simulink model "model2_unstable__lqr_controller_observer"  (R2022b)
settings: Solver=VariableStepAuto  StartTime=0.0  StopTime=10  RelTol=1e-3
InitFcn:
  | model2_init_params_unstable__lqr_controller
values from neighbouring files (symbols this model uses):
  A = [ ... (first row only)    [model1_init_params_stable.m]    (also in model1_init_params_unstable.m; model2_init_params_stable.m; model2_init_params_unstable.m; model2_init_params_unstable__lqr_controller.m)
  A_ccf = [ ... (first row only)    [model2_init_params_stable.m]    (also in model2_init_params_unstable.m; model2_init_params_unstable__lqr_controller.m)
  A_obs = A-L*C    [model1_init_params_stable.m]    (also in model1_init_params_unstable.m; model2_init_params_unstable__lqr_controller.m = A_ccf-L*C_ccf)
  B = [ ... (first row only)    [model1_init_params_stable.m]    (also in model1_init_params_unstable.m; model2_init_params_stable.m; model2_init_params_unstable.m; model2_init_params_unstable__lqr_controller.m)
  B_obs = [B L]    [model1_init_params_stable.m]    (also in model1_init_params_unstable.m; model2_init_params_unstable__lqr_controller.m = [B_ccf L])
  C = [(V^2*h-a*c*g)*sin(lambda)/(b*h^2)*k1 a*V*sin(lambda)/(b*h)*k1]    [model1_init_params_stable.m]    (also in model1_init_params_unstable.m; model2_init_params_stable.m = [1 0 0 0]; model2_init_params_unstable.m = [1 0 0 0]; model2_init_params_unstable__lqr_controller.m = [1 0 0 0])
  C_ccf = [tf_num(5)  tf_num(4)   tf_num(3)   tf_num(2)]    [model2_init_params_stable.m]    (also in model2_init_params_unstable.m; model2_init_params_unstable__lqr_controller.m)
  C_obs = eye(length(A_obs))    [model1_init_params_stable.m]    (also in model1_init_params_unstable.m; model2_init_params_unstable__lqr_controller.m)
  D = 0    [model1_init_params_stable.m]    (also in model1_init_params_unstable.m; model2_init_params_stable.m; model2_init_params_unstable.m; model2_init_params_unstable__lqr_controller.m)
  D_obs = zeros(size(B_obs))    [model1_init_params_stable.m]    (also in model1_init_params_unstable.m; model2_init_params_unstable__lqr_controller.m)
  K = place(A,B,new_poles)    [model1_init_params_unstable.m]    (also in model2_init_params_unstable.m = place(A_ccf,B_ccf,new_poles))
settings Model: Creator=neotod  LastModifiedBy=neotod

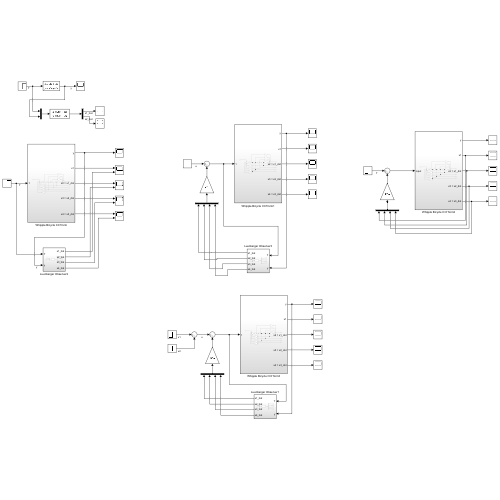
[thumbnail: Simulink's stored preview of the top-level diagram]
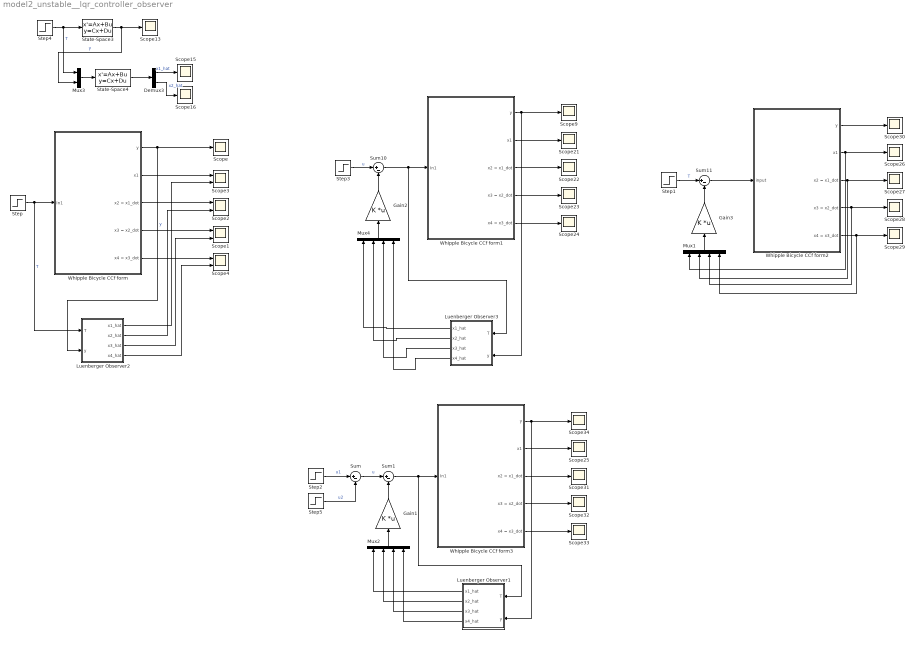
== system model2_unstable__lqr_controller_observer ==
  Demux3 : Demux  Outputs=2
  Gain1 : Gain  Gain=K  Multiplication=Matrix(K*u)
  Gain2 : Gain  Gain=K  Multiplication=Matrix(K*u)
  Gain3 : Gain  Gain=K  Multiplication=Matrix(K*u)
  Luenberger Observer1 : Subsystem
  Luenberger Observer2 : Subsystem
  Luenberger Observer3 : Subsystem
  Mux1 : Mux
  Mux2 : Mux
  Mux3 : Mux  Inputs=2
  Mux4 : Mux
  Scope{,9,13,15..16,21..34} (19 alike) : Scope
  Scope{1..4} (4 alike) : Scope  NumInputPorts=2
  State-Space3 : StateSpace  A=A  B=B  C=C  D=D  InitialCondition=0
  State-Space4 : StateSpace  A=A_obs  B=B_obs  C=C_obs  D=D_obs  InitialCondition=0
  Step : Step  After=0.6  SampleTime=0
  Step1 : Step  After=0.6  SampleTime=0
  Step2 : Step  Time=0.25  SampleTime=0
  Step3 : Step  After=0.6  SampleTime=0
  Step4 : Step  SampleTime=0
  Step5 : Step  Time=0.5  SampleTime=0
  Sum{,1,10..11} (4 alike) : Sum  Inputs=|+-
  Whipple Bicycle CCf form : Subsystem
  Whipple Bicycle CCf form1 : Subsystem
  Whipple Bicycle CCf form2 : Subsystem
  Whipple Bicycle CCf form3 : Subsystem
  wires:
  Step4/1 -> Mux3/1, State-Space3/1  "T"
  State-Space3/1 -> Mux3/2, Scope13/1  "y"
  State-Space4/1 -> Demux3/1
  Mux3/1 -> State-Space4/1
  Demux3/1 -> Scope15/1  "x1_hat"
  Demux3/2 -> Scope16/1  "x2_hat"
  Whipple Bicycle CCf form/2(x1) -> Scope3/1
  Whipple Bicycle CCf form/5(x4 = x3_dot) -> Scope4/1
  Whipple Bicycle CCf form/4(x3 = x2_dot) -> Scope1/1
  Whipple Bicycle CCf form/3(x2 = x1_dot) -> Scope2/1
  Step/1 -> Luenberger Observer2/1(T), Whipple Bicycle CCf form/1(In1)  "T"
  Whipple Bicycle CCf form/1(y) -> Luenberger Observer2/2(y), Scope/1  "y"
  Whipple Bicycle CCf form1/5(x4 = x3_dot) -> Scope24/1
  Luenberger Observer3/2(x2_hat) -> Mux4/2
  Whipple Bicycle CCf form1/4(x3 = x2_dot) -> Scope23/1
  Luenberger Observer3/3(x3_hat) -> Mux4/3
  Whipple Bicycle CCf form1/2(x1) -> Scope21/1
  Whipple Bicycle CCf form1/3(x2 = x1_dot) -> Scope22/1
  Luenberger Observer3/1(x1_hat) -> Mux4/1
  Luenberger Observer3/4(x4_hat) -> Mux4/4
  Whipple Bicycle CCf form1/1(y) -> Luenberger Observer3/2(y), Scope9/1
  Step3/1 -> Sum10/1  "u"
  Sum10/1 -> Luenberger Observer3/1(T), Whipple Bicycle CCf form1/1(In1)
  Mux4/1 -> Gain2/1
  Gain2/1 -> Sum10/2
  Sum11/1 -> Whipple Bicycle CCf form2/1(input)
  Step1/1 -> Sum11/1  "T"
  Whipple Bicycle CCf form2/2(x1) -> Mux1/1, Scope26/1
  Whipple Bicycle CCf form2/3(x2 = x1_dot) -> Mux1/2, Scope27/1
  Whipple Bicycle CCf form2/5(x4 = x3_dot) -> Mux1/4, Scope29/1
  Mux1/1 -> Gain3/1
  Gain3/1 -> Sum11/2
  Whipple Bicycle CCf form2/4(x3 = x2_dot) -> Mux1/3, Scope28/1
  Whipple Bicycle CCf form2/1(y) -> Scope30/1
  Sum1/1 -> Luenberger Observer1/1(T), Whipple Bicycle CCf form3/1(In1)
  Gain1/1 -> Sum1/2
  Whipple Bicycle CCf form3/4(x3 = x2_dot) -> Scope32/1
  Whipple Bicycle CCf form3/3(x2 = x1_dot) -> Scope31/1
  Whipple Bicycle CCf form3/1(y) -> Luenberger Observer1/2(y), Scope34/1
  Mux2/1 -> Gain1/1
  Luenberger Observer1/4(x4_hat) -> Mux2/4
  Luenberger Observer1/1(x1_hat) -> Mux2/1
  Whipple Bicycle CCf form3/5(x4 = x3_dot) -> Scope33/1
  Luenberger Observer1/2(x2_hat) -> Mux2/2
  Luenberger Observer1/3(x3_hat) -> Mux2/3
  Whipple Bicycle CCf form3/2(x1) -> Scope25/1
  Sum/1 -> Sum1/1  "u"
  Step2/1 -> Sum/1  "u1"
  Step5/1 -> Sum/2  "u2"
  Luenberger Observer2/1(x1_hat) -> Scope3/2
  Luenberger Observer2/2(x2_hat) -> Scope2/2
  Luenberger Observer2/3(x3_hat) -> Scope1/2
  Luenberger Observer2/4(x4_hat) -> Scope4/2

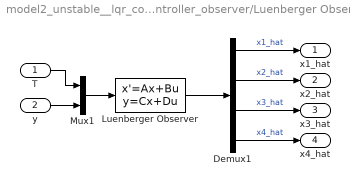
== system model2_unstable__lqr_controller_observer/Luenberger Observer1 ==
  T : Inport
  y : Inport  Port=2
  Demux1 : Demux
  Luenberger Observer : StateSpace  A=A_obs  B=B_obs  C=C_obs  D=D_obs  InitialCondition=0
  Mux1 : Mux  Inputs=2
  x1_hat : Outport
  x2_hat : Outport  Port=2
  x3_hat : Outport  Port=3
  x4_hat : Outport  Port=4
  wires:
  Demux1/2 -> x2_hat/1  "x2_hat"
  Mux1/1 -> Luenberger Observer/1
  Luenberger Observer/1 -> Demux1/1
  Demux1/1 -> x1_hat/1  "x1_hat"
  Demux1/3 -> x3_hat/1  "x3_hat"
  Demux1/4 -> x4_hat/1  "x4_hat"
  y/1 -> Mux1/2
  T/1 -> Mux1/1

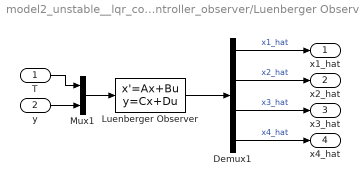
== system model2_unstable__lqr_controller_observer/Luenberger Observer2 ==
  T : Inport
  y : Inport  Port=2
  Demux1 : Demux
  Luenberger Observer : StateSpace  A=A_obs  B=B_obs  C=C_obs  D=D_obs  InitialCondition=0
  Mux1 : Mux  Inputs=2
  x1_hat : Outport
  x2_hat : Outport  Port=2
  x3_hat : Outport  Port=3
  x4_hat : Outport  Port=4
  wires:
  Demux1/2 -> x2_hat/1  "x2_hat"
  Mux1/1 -> Luenberger Observer/1
  Luenberger Observer/1 -> Demux1/1
  Demux1/1 -> x1_hat/1  "x1_hat"
  Demux1/3 -> x3_hat/1  "x3_hat"
  Demux1/4 -> x4_hat/1  "x4_hat"
  T/1 -> Mux1/1
  y/1 -> Mux1/2

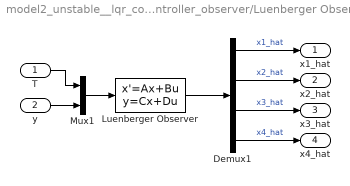
== system model2_unstable__lqr_controller_observer/Luenberger Observer3 ==
  T : Inport
  y : Inport  Port=2
  Demux1 : Demux
  Luenberger Observer : StateSpace  A=A_obs  B=B_obs  C=C_obs  D=D_obs  InitialCondition=0
  Mux1 : Mux  Inputs=2
  x1_hat : Outport
  x2_hat : Outport  Port=2
  x3_hat : Outport  Port=3
  x4_hat : Outport  Port=4
  wires:
  Demux1/2 -> x2_hat/1  "x2_hat"
  Mux1/1 -> Luenberger Observer/1
  Luenberger Observer/1 -> Demux1/1
  Demux1/1 -> x1_hat/1  "x1_hat"
  Demux1/3 -> x3_hat/1  "x3_hat"
  Demux1/4 -> x4_hat/1  "x4_hat"
  y/1 -> Mux1/2
  T/1 -> Mux1/1

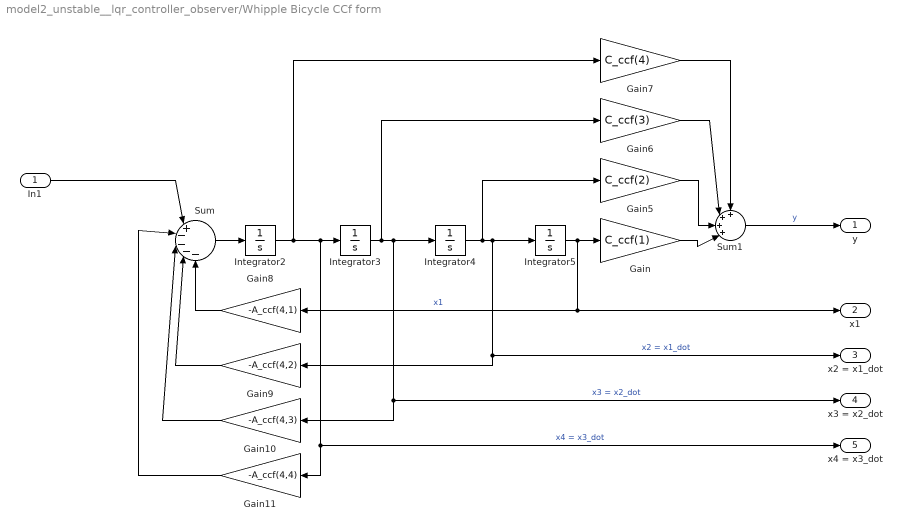
== system model2_unstable__lqr_controller_observer/Whipple Bicycle CCf form ==
  In1 : Inport
  Gain : Gain  Gain=C_ccf(1)
  Gain10 : Gain  Gain=-A_ccf(4,3)
  Gain11 : Gain  Gain=-A_ccf(4,4)
  Gain5 : Gain  Gain=C_ccf(2)
  Gain6 : Gain  Gain=C_ccf(3)
  Gain7 : Gain  Gain=C_ccf(4)
  Gain8 : Gain  Gain=-A_ccf(4,1)
  Gain9 : Gain  Gain=-A_ccf(4,2)
  Integrator{2..5} (4 alike) : Integrator
  Sum : Sum  Inputs=|+----
  Sum1 : Sum  Inputs=++++|
  y : Outport
  x1 : Outport  Port=2
  x2 = x1_dot : Outport  Port=3
  x3 = x2_dot : Outport  Port=4
  x4 = x3_dot : Outport  Port=5
  wires:
  Integrator3/1 -> Gain6/1, x3 = x2_dot/1, Gain10/1, Integrator4/1  "x3 = x2_dot"
  Gain7/1 -> Sum1/1
  Integrator2/1 -> Gain7/1, x4 = x3_dot/1, Gain11/1, Integrator3/1  "x4 = x3_dot"
  Integrator5/1 -> x1/1, Gain8/1, Gain/1  "x1"
  Gain10/1 -> Sum/3
  Integrator4/1 -> Gain5/1, x2 = x1_dot/1, Gain9/1, Integrator5/1  "x2 = x1_dot"
  Gain6/1 -> Sum1/2
  Sum1/1 -> y/1  "y"
  In1/1 -> Sum/1
  Gain8/1 -> Sum/5
  Sum/1 -> Integrator2/1
  Gain5/1 -> Sum1/3
  Gain/1 -> Sum1/4
  Gain11/1 -> Sum/2
  Gain9/1 -> Sum/4

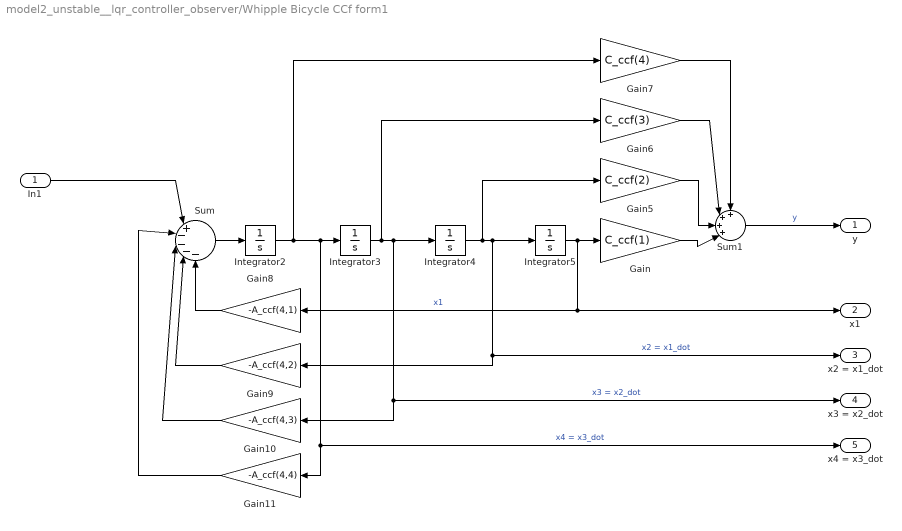
== system model2_unstable__lqr_controller_observer/Whipple Bicycle CCf form1 ==
  In1 : Inport
  Gain : Gain  Gain=C_ccf(1)
  Gain10 : Gain  Gain=-A_ccf(4,3)
  Gain11 : Gain  Gain=-A_ccf(4,4)
  Gain5 : Gain  Gain=C_ccf(2)
  Gain6 : Gain  Gain=C_ccf(3)
  Gain7 : Gain  Gain=C_ccf(4)
  Gain8 : Gain  Gain=-A_ccf(4,1)
  Gain9 : Gain  Gain=-A_ccf(4,2)
  Integrator{2..5} (4 alike) : Integrator
  Sum : Sum  Inputs=|+----
  Sum1 : Sum  Inputs=++++|
  y : Outport
  x1 : Outport  Port=2
  x2 = x1_dot : Outport  Port=3
  x3 = x2_dot : Outport  Port=4
  x4 = x3_dot : Outport  Port=5
  wires:
  Integrator3/1 -> Gain6/1, x3 = x2_dot/1, Gain10/1, Integrator4/1  "x3 = x2_dot"
  Gain7/1 -> Sum1/1
  Integrator2/1 -> Gain7/1, x4 = x3_dot/1, Gain11/1, Integrator3/1  "x4 = x3_dot"
  Integrator5/1 -> x1/1, Gain8/1, Gain/1  "x1"
  Gain10/1 -> Sum/3
  Integrator4/1 -> Gain5/1, x2 = x1_dot/1, Gain9/1, Integrator5/1  "x2 = x1_dot"
  Gain6/1 -> Sum1/2
  Sum1/1 -> y/1  "y"
  In1/1 -> Sum/1
  Gain8/1 -> Sum/5
  Sum/1 -> Integrator2/1
  Gain5/1 -> Sum1/3
  Gain/1 -> Sum1/4
  Gain11/1 -> Sum/2
  Gain9/1 -> Sum/4

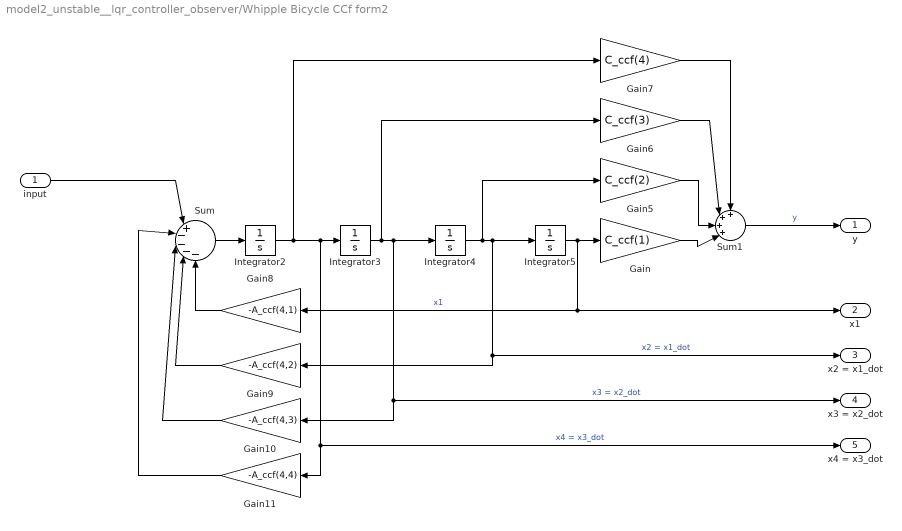
== system model2_unstable__lqr_controller_observer/Whipple Bicycle CCf form2 ==
  input : Inport
  Gain : Gain  Gain=C_ccf(1)
  Gain10 : Gain  Gain=-A_ccf(4,3)
  Gain11 : Gain  Gain=-A_ccf(4,4)
  Gain5 : Gain  Gain=C_ccf(2)
  Gain6 : Gain  Gain=C_ccf(3)
  Gain7 : Gain  Gain=C_ccf(4)
  Gain8 : Gain  Gain=-A_ccf(4,1)
  Gain9 : Gain  Gain=-A_ccf(4,2)
  Integrator{2..5} (4 alike) : Integrator
  Sum : Sum  Inputs=|+----
  Sum1 : Sum  Inputs=++++|
  y : Outport
  x1 : Outport  Port=2
  x2 = x1_dot : Outport  Port=3
  x3 = x2_dot : Outport  Port=4
  x4 = x3_dot : Outport  Port=5
  wires:
  Integrator3/1 -> Gain6/1, x3 = x2_dot/1, Gain10/1, Integrator4/1  "x3 = x2_dot"
  Gain7/1 -> Sum1/1
  Integrator2/1 -> Gain7/1, x4 = x3_dot/1, Gain11/1, Integrator3/1  "x4 = x3_dot"
  Integrator5/1 -> x1/1, Gain8/1, Gain/1  "x1"
  Gain10/1 -> Sum/3
  Integrator4/1 -> Gain5/1, x2 = x1_dot/1, Gain9/1, Integrator5/1  "x2 = x1_dot"
  Gain6/1 -> Sum1/2
  Sum1/1 -> y/1  "y"
  input/1 -> Sum/1
  Gain8/1 -> Sum/5
  Sum/1 -> Integrator2/1
  Gain5/1 -> Sum1/3
  Gain/1 -> Sum1/4
  Gain11/1 -> Sum/2
  Gain9/1 -> Sum/4

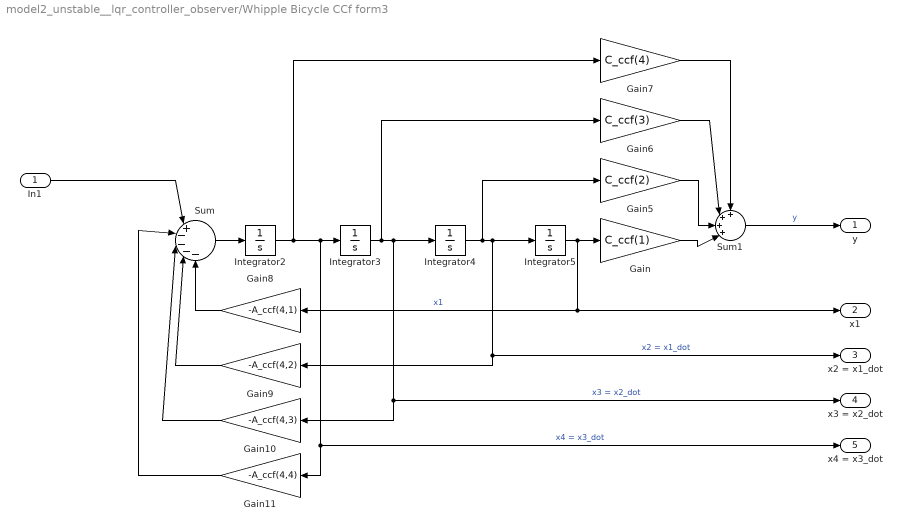
== system model2_unstable__lqr_controller_observer/Whipple Bicycle CCf form3 ==
  In1 : Inport
  Gain : Gain  Gain=C_ccf(1)
  Gain10 : Gain  Gain=-A_ccf(4,3)
  Gain11 : Gain  Gain=-A_ccf(4,4)
  Gain5 : Gain  Gain=C_ccf(2)
  Gain6 : Gain  Gain=C_ccf(3)
  Gain7 : Gain  Gain=C_ccf(4)
  Gain8 : Gain  Gain=-A_ccf(4,1)
  Gain9 : Gain  Gain=-A_ccf(4,2)
  Integrator{2..5} (4 alike) : Integrator
  Sum : Sum  Inputs=|+----
  Sum1 : Sum  Inputs=++++|
  y : Outport
  x1 : Outport  Port=2
  x2 = x1_dot : Outport  Port=3
  x3 = x2_dot : Outport  Port=4
  x4 = x3_dot : Outport  Port=5
  wires:
  Integrator3/1 -> Gain6/1, x3 = x2_dot/1, Gain10/1, Integrator4/1  "x3 = x2_dot"
  Gain7/1 -> Sum1/1
  Integrator2/1 -> Gain7/1, x4 = x3_dot/1, Gain11/1, Integrator3/1  "x4 = x3_dot"
  Integrator5/1 -> x1/1, Gain8/1, Gain/1  "x1"
  Gain10/1 -> Sum/3
  Integrator4/1 -> Gain5/1, x2 = x1_dot/1, Gain9/1, Integrator5/1  "x2 = x1_dot"
  Gain6/1 -> Sum1/2
  Sum1/1 -> y/1  "y"
  In1/1 -> Sum/1
  Gain8/1 -> Sum/5
  Sum/1 -> Integrator2/1
  Gain5/1 -> Sum1/3
  Gain/1 -> Sum1/4
  Gain11/1 -> Sum/2
  Gain9/1 -> Sum/4
